simulink model "simulink_first"  (R2015b)
settings: Solver=VariableStepAuto  StartTime=0.0  StopTime=4000  RelTol=1e-3
values from neighbouring files (symbols this model uses):
  a_m = sys_M.A    [Matlab_exam.m]
  A_p = sys_G.A    [Matlab_exam.m]
  b_m = sys_M.B    [Matlab_exam.m]
  B_p = sys_G.B    [Matlab_exam.m]
  c_m = sys_M.C    [Matlab_exam.m]
  C_p = sys_G.C    [Matlab_exam.m]
  d_m = sys_M.D    [Matlab_exam.m]
  D_p = sys_G.D    [Matlab_exam.m]
  Gamma = eye(2*n).*100    [Matlab_exam.m]    (also in Matlab_uppg3.m = eye(2).*3)
  k_p = 1    [Matlab_exam.m]
  l = sys_F.B    [Matlab_exam.m]
  Lambda = sys_F.A    [Matlab_exam.m]
  param_init = zeros(2*n,1)    [Matlab_exam.m]
  phi_1_init = zeros(n-1,1)    [Matlab_exam.m]
  phi_2_init = zeros(n-1,1)    [Matlab_exam.m]
  x_m_init = zeros(n,1)    [Matlab_exam.m]
  x_p_init = zeros(n,1)    [Matlab_exam.m]
settings Model: Creator=Albin  LastModifiedBy=Albin

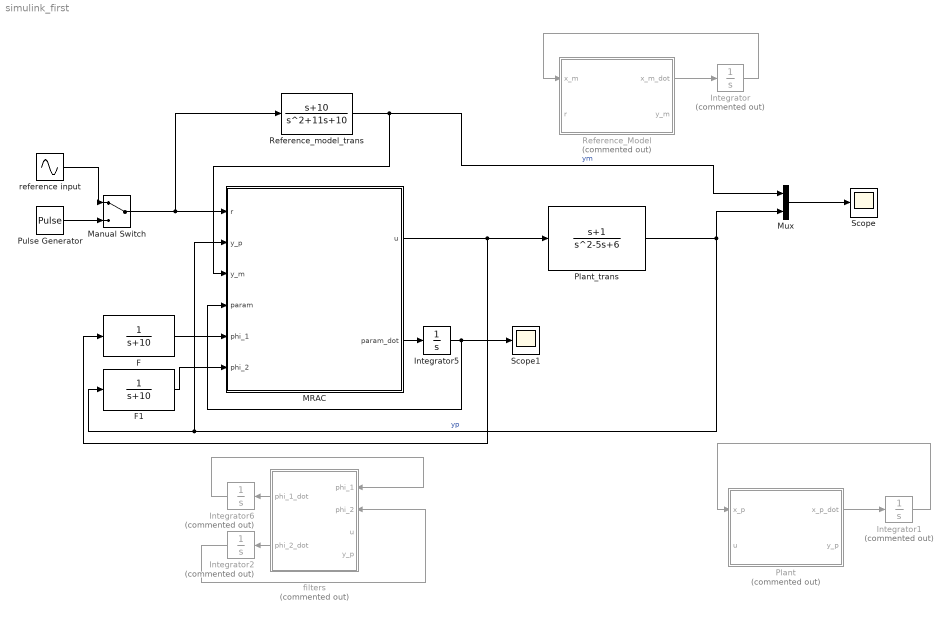
== system simulink_first ==
  F : TransferFcn  Denominator=[1 10]
  F1 : TransferFcn  Denominator=[1 10]
  Integrator : Integrator  Commented=on  InitialCondition=x_m_init
  Integrator1 : Integrator  Commented=on  InitialCondition=x_p_init
  Integrator2 : Integrator  Commented=on  InitialCondition=phi_2_init
  Integrator5 : Integrator  InitialCondition=param_init
  Integrator6 : Integrator  Commented=on  InitialCondition=phi_1_init
  MRAC : MATLAB Function  TreatAsAtomicUnit=on
  Manual Switch : ManualSwitch
  Mux : Mux  Inputs=2
  Plant : MATLAB Function  Commented=on  TreatAsAtomicUnit=on
  Plant_trans : TransferFcn  Numerator=[1 1]  Denominator=[1 -5 +6]
  Pulse Generator : DiscretePulseGenerator  PulseType=Time based  Amplitude=4  Period=20  PulseWidth=50
  Reference_Model : MATLAB Function  Commented=on  TreatAsAtomicUnit=on
  Reference_model_trans : TransferFcn  Numerator=[1 10]  Denominator=[1 11 10]
  Scope : Scope
  Scope1 : Scope
  filters : MATLAB Function  Commented=on  TreatAsAtomicUnit=on
  reference input : Sin  Amplitude=4  Frequency=4  SampleTime=0
  wires:
  Plant/1(x_p_dot) -> Integrator1/1
  Reference_Model/1(x_m_dot) -> Integrator/1
  Integrator/1 -> Reference_Model/1(x_m)
  Integrator1/1 -> Plant/1(x_p)
  MRAC/2(param_dot) -> Integrator5/1
  Integrator5/1 -> MRAC/4(param), Scope1/1
  Mux/1 -> Scope/1
  filters/1(phi_1_dot) -> Integrator6/1
  filters/2(phi_2_dot) -> Integrator2/1
  Integrator6/1 -> filters/1(phi_1)
  Integrator2/1 -> filters/2(phi_2)
  Pulse Generator/1 -> Manual Switch/2
  Manual Switch/1 -> Reference_model_trans/1, MRAC/1(r)
  reference input/1 -> Manual Switch/1
  MRAC/1(u) -> Plant_trans/1, F/1
  Plant_trans/1 -> F1/1, MRAC/2(y_p), Mux/2  "yp"
  Reference_model_trans/1 -> MRAC/3(y_m), Mux/1  "ym"
  F/1 -> MRAC/5(phi_1)
  F1/1 -> MRAC/6(phi_2)

== matlab function simulink_first/Reference_Model ==
  data: x_m input; x_m_dot output; r input; a_m parameter; b_m parameter; y_m output; c_m parameter; d_m parameter
function [x_m_dot,y_m] = fcn(x_m,r,a_m,b_m,c_m,d_m)
%#Reference model for the MRAC

x_m_dot = a_m*x_m + b_m*r;
y_m = c_m*x_m + d_m*r;

== matlab function simulink_first/Plant ==
  data: x_p input; u input; x_p_dot output; y_p output; A_p parameter; B_p parameter; C_p parameter; D_p parameter
function [x_p_dot,y_p] = fcn(x_p,u,A_p,B_p,C_p,D_p)
%#Plant model

x_p_dot = A_p*x_p + B_p*u;
y_p = C_p*x_p + D_p*u;

== matlab function simulink_first/MRAC ==
  data: r input; y_p input; y_m input; Gamma parameter; param input; k_p parameter; u output; phi_1 input; phi_2 input; param_dot output
function [u,param_dot]  = fcn(r,y_p,y_m,Gamma,param,k_p,phi_1,phi_2)

% Error 
error = y_p - y_m;      % Error between the states

% Parameter estimation with regressor
phi = [r,phi_1',y_p,phi_2']';

% Regressor
param_dot = -sign(k_p).*error.*Gamma*phi;       % Adaptive parameter law

%Adaptive control law
u = param'*phi;

== matlab function simulink_first/filters ==
  data: phi_1 input; phi_2 input; u input; phi_1_dot output; y_p input; Lambda parameter; l parameter; phi_2_dot output
function [phi_1_dot,phi_2_dot] = fcn(phi_1,phi_2,u,y_p,Lambda,l)
%#codegen

phi_1_dot = Lambda*phi_1 + l*u;            % Feed forward filter
phi_2_dot = Lambda*phi_2 + l*y_p;          % Output feedback filter
